simulink model "LOC_SYSTEM_20112024_2_Model"  (R2024a)
settings: Solver=VariableStepAuto  StartTime=0.0  StopTime=10.0  FixedStep=0.001  RelTol=1e-3
undefined symbols (not defined in the file): cp_oil, cp_water, engine_max_load, HE_heat_transfer_coefficient, HE_m1, HE_m2, HE_surface_area, HE_T1_ini, HE_T2_ini, LO_cooling_mass_oil_side, LO_cooling_mass_water_side, LO_heat_transfer_coefficient, LO_initial_temperatures
settings Model: ExtModeTrigDuration=100  Creator=ojklem  LastModifiedBy=ojklem
settings DataIOCC: StateSaveName=tmp_raccel_xout
settings OptimizationCC: EfficientMapNaN2IntZero=off
settings RTWCC: CustomBLASCallback=coder.internal.blas.MATLABBLASCallback
settings CodeAppCC: GenerateComments=off  MangleLength=10  SimulinkBlockComments=off

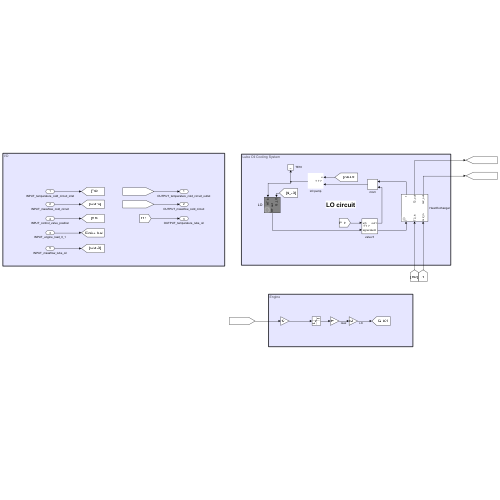
[thumbnail: Simulink's stored preview of the top-level diagram]
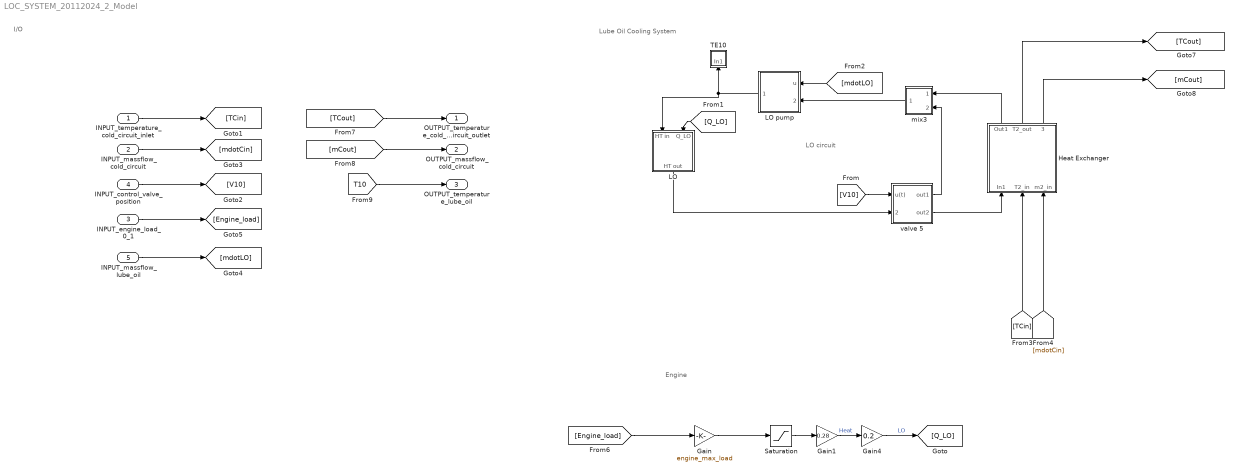
== system LOC_SYSTEM_20112024_2_Model ==
  note: LO circuit
  note: Lube Oil Cooling System
  note: Engine
  note: I/O
  INPUT_temperature_cold_circuit_inlet : Inport
  INPUT_massflow_cold_circuit : Inport  Port=2
  INPUT_engine_load_0_1 : Inport  Port=3
  INPUT_control_valve_position : Inport  Port=4
  INPUT_massflow_lube_oil : Inport  Port=5
  Gain : Gain  Gain=engine_max_load
  Gain1 : Gain  Gain=0.28
  Gain4 : Gain  Gain=0.2
  Heat Exchanger : Subsystem  mask{m1=HE_m1, m2=HE_m2, cp1=cp_water, cp2=cp_water, Tini=[HE_T1_ini, HE_T2_ini], A=HE_surface_area, h=HE_heat_transfer_coefficient}
      mask prompts: m1 "Mass side 1"; m2 "Mass side 2"; cp1 "Heat capacity side 1"; cp2 "Heat capacity side 2"; Tini "Initial value"; A "Area"; h "Heat transfer coefficient"
  LO : Subsystem  mask{K=LO_heat_transfer_coefficient, cpC=cp_water, cpSteel=cp_oil, MC=LO_cooling_mass_water_side, MSteel=LO_cooling_mass_oil_side, InitT=[LO_initial_temperatures, LO_initial_temperatures]}
      mask prompts: K "Heat transfer coefficient:"; cpC "Specific heat capacity water [J/kgK]:"; cpSteel "Specific heat capacity LO: [J/kgK]"; MC "Mass water [kg]:"; MSteel "Mass LO [kg]:"; InitT "Initial temperatures:"
  LO pump : Subsystem
      mask Display: image('pump.jpg');
  Saturation : Saturate  UpperLimit=engine_max_load  LowerLimit=0
  TE10 : Subsystem
  mix3 : Subsystem
      mask Display: % image('mix.png')
  valve 5 : Subsystem
      mask Display: image('valve3.png')
  OUTPUT_temperature_cold_circuit_outlet : Outport
  OUTPUT_massflow_cold_circuit : Outport  Port=2
  OUTPUT_temperature_lube_oil : Outport  Port=3
  wires:
  LO pump/1("  ") -> LO/1(HT in), TE10/1(In1)
  mix3/1(Out1) -> LO pump/2(" ")
  [mdotLO] -> LO pump/1(u)
  [mdotCin] -> Heat Exchanger/3(m2_in)
  [V10] -> valve 5/1(u(t))
  [TCin] -> Heat Exchanger/2(T2_in)
  Heat Exchanger/2(T2_out) -> [TCout]
  Heat Exchanger/1(Out1) -> mix3/1(In1)
  LO/1(HT out) -> valve 5/2(signal in)
  [Q_LO] -> LO/2(Q_LO)
  valve 5/2("out2 ") -> Heat Exchanger/1(In1)
  Heat Exchanger/3(m2_out) -> [mCout]
  valve 5/1(out1) -> mix3/2(In2)
  Gain1/1 -> Gain4/1  "Heat"
  Gain/1 -> Saturation/1
  [Engine_load] -> Gain/1
  Gain4/1 -> [Q_LO]  "LO"
  Saturation/1 -> Gain1/1
  [TCout] -> OUTPUT_temperature_cold_circuit_outlet/1
  INPUT_engine_load_0_1/1 -> [Engine_load]
  INPUT_massflow_cold_circuit/1 -> [mdotCin]
  INPUT_temperature_cold_circuit_inlet/1 -> [TCin]
  [mCout] -> OUTPUT_massflow_cold_circuit/1
  [T10] -> OUTPUT_temperature_lube_oil/1
  INPUT_control_valve_position/1 -> [V10]
  INPUT_massflow_lube_oil/1 -> [mdotLO]

== system LOC_SYSTEM_20112024_2_Model/Heat Exchanger ==
  In1 : Inport
  T2_in : Inport  Port=2
  m2_in : Inport  Port=3
  Demux : Demux  Outputs=2
  HX : Subsystem
      settings: PortSchema="{\"entries\":[{\"content\":{\"sides\":[{\"content\":{\"connectorIds\":[\"Out1\",\"Out2\",\"Out3\",\"Out4\"]},\"type\":\"ConnectorPlacement.EquallySpacedRectSide\",\"uuid\":\"b608803e-13f5-49cd-ab3a-92503d47ac52\"},{\"content\":{\"connectorIds\":[\"In1\",\"In2\",\"In3\",\"In4\"],\"side\":\"RIGHT\"},\"type\":\"ConnectorPlacement.EquallySpacedRectSide\",\"uuid\":\"cb859c45-d915-447d-9a89-62abad3e0c6f\"},{\"content\":{\"side\":\"TOP\"},\"type\":\"ConnectorPlacement.EquallySpacedRectSide\",\"uuid\":\"d365d95d-a075-458d-ace5-a17a7cf71809\"}]},\"type\":\"ConnectorPlacement.EquallySpacedConnector\",\"uuid\":\"ca673d01-47a6-46be-9ba4-be473b696b68\"}],\"packageUris\":[\"http://schema.mathworks.com/mf0/Connector/R2020b\"],\"version\":\"1.0\"}"
  Mux : Mux  Inputs=2
  Out1 : Outport
  T2_out : Outport  Port=2
  m2_out : Outport  Port=3
  wires:
  Demux/1 -> HX/4(T1_in)
  HX/4(T1_out) -> Mux/1
  Demux/2 -> HX/3(m1_in)
  HX/3(m1_out) -> Mux/2
  HX/1(m2_out) -> m2_out/1
  In1/1 -> Demux/1
  Mux/1 -> Out1/1
  T2_in/1 -> HX/2(T2_in)
  m2_in/1 -> HX/1(m2_in)
  HX/2(T2_out) -> T2_out/1

== system LOC_SYSTEM_20112024_2_Model/LO ==
  HT in : Inport
  Q_LO : Inport  Port=2
  Demux : Demux  Outputs=2
  Mux1 : Mux  Inputs=2
  Scope : Scope
  Subsystem : Subsystem
  Transport Delay : TransportDelay  Commented=on  DelayTime=0.2*60  InitialOutput=40
  Variable time-delay10 : Subsystem  Commented=on  mask{PipeVolume=MC/1000, InitOut=InitT(2)}
      mask prompts: PipeVolume "Pipe Volume [m^3]:"; InitOut "Initial Output:"
  HT out : Outport  VectorParamsAs1DForOutWhenUnconnected=off
  wires:
  Q_LO/1 -> Subsystem/3(Q)
  HT in/1 -> Demux/1
  Demux/2 -> Subsystem/2(m)
  Demux/1 -> Subsystem/1(Tin)
  Subsystem/3(m2) -> Mux1/2
  Subsystem/2(T) -> Scope/1
  Subsystem/1(Tout) -> Mux1/1
  Mux1/1 -> HT out/1

== system LOC_SYSTEM_20112024_2_Model/LO pump ==
  u : Inport
  " " : Inport  Port=2
  Demux : Demux  Outputs=2
  Mux8 : Mux  Inputs=2
  Scope : Scope
  "  " : Outport  VectorParamsAs1DForOutWhenUnconnected=off
  wires:
  " "/1 -> Demux/1
  Mux8/1 -> "  "/1
  u/1 -> Mux8/2
  Demux/2 -> Scope/1
  Demux/1 -> Mux8/1

== system LOC_SYSTEM_20112024_2_Model/TE10 ==
  In1 : Inport
  Gain : Gain  Gain=[1 0]  Multiplication=Matrix(K*u)
  tag scope: T10=global
  wires:
  Gain/1 -> [T10]
  In1/1 -> Gain/1

== system LOC_SYSTEM_20112024_2_Model/mix3 ==
  In1 : Inport
  In2 : Inport  Port=2
  Fcn : Fcn  Expr=(u(1)*u(2) + u(3)*u(4))/( u(2)+u(4) )
  Fcn1 : Fcn  Expr=u(2)+u(4)
  Mux1 : Mux  Inputs=2
  Mux2 : Mux  Inputs=2
  Scope1 : Scope
  Scope2 : Scope
  Out1 : Outport  VectorParamsAs1DForOutWhenUnconnected=off
  wires:
  In1/1 -> Scope1/1, Mux1/1
  Mux2/1 -> Out1/1
  In2/1 -> Mux1/2
  Fcn/1 -> Mux2/1
  Mux1/1 -> Fcn1/1, Scope2/1, Fcn/1
  Fcn1/1 -> Mux2/2

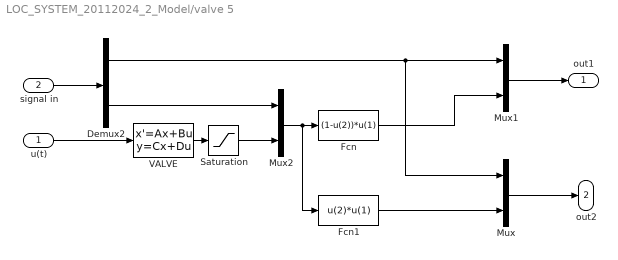
== system LOC_SYSTEM_20112024_2_Model/valve 5 ==
  u(t) : Inport
  signal in : Inport  Port=2
  Demux2 : Demux  Outputs=2
  Fcn : Fcn  Expr=(1-u(2))*u(1)
  Fcn1 : Fcn  Expr=u(2)*u(1)
  Mux : Mux  Inputs=2
  Mux1 : Mux  Inputs=2
  Mux2 : Mux  Inputs=2
  Saturation : Saturate  UpperLimit=0.99  LowerLimit=0.01
  VALVE : StateSpace  A=-1/1  B=1/1  D=0  InitialCondition=1
  out1 : Outport  VectorParamsAs1DForOutWhenUnconnected=off
  "out2 " : Outport  Port=2  VectorParamsAs1DForOutWhenUnconnected=off
  wires:
  Mux/1 -> "out2 "/1
  signal in/1 -> Demux2/1
  Mux1/1 -> out1/1
  Demux2/1 -> Mux/1, Mux1/1
  Mux2/1 -> Fcn1/1, Fcn/1
  Fcn/1 -> Mux1/2
  Fcn1/1 -> Mux/2
  VALVE/1 -> Saturation/1
  Demux2/2 -> Mux2/1
  u(t)/1 -> VALVE/1
  Saturation/1 -> Mux2/2

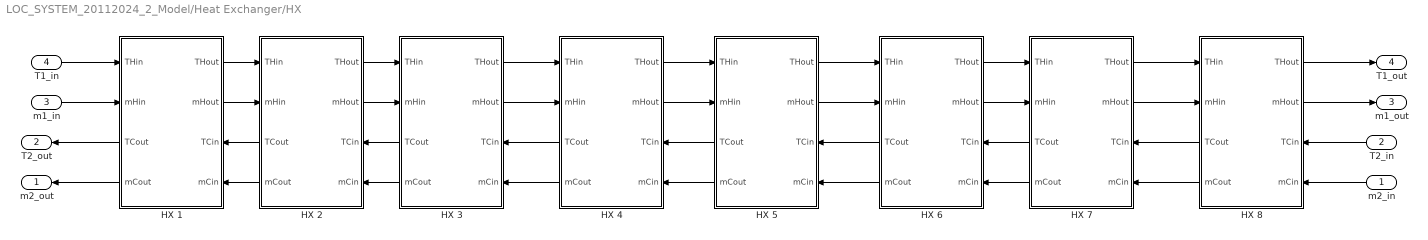
== system LOC_SYSTEM_20112024_2_Model/Heat Exchanger/HX ==
  m2_in : Inport
  T2_in : Inport  Port=2
  m1_in : Inport  Port=3
  T1_in : Inport  Port=4
  HX 1 : Subsystem
      settings: PortSchema="{\"entries\":[{\"content\":{\"sides\":[{\"content\":{\"connectorIds\":[\"In1\",\"In2\",\"Out3\",\"Out4\"]},\"type\":\"ConnectorPlacement.EquallySpacedRectSide\",\"uuid\":\"b608803e-13f5-49cd-ab3a-92503d47ac52\"},{\"content\":{\"connectorIds\":[\"Out1\",\"Out2\",\"In3\",\"In4\"],\"side\":\"RIGHT\"},\"type\":\"ConnectorPlacement.EquallySpacedRectSide\",\"uuid\":\"cb859c45-d915-447d-9a89-62abad3e0c6f\"},{\"content\":{\"connectorIds\":[],\"side\":\"TOP\"},\"type\":\"ConnectorPlacement.EquallySpacedRectSide\",\"uuid\":\"d365d95d-a075-458d-ace5-a17a7cf71809\"}]},\"type\":\"ConnectorPlacement.EquallySpacedConnector\",\"uuid\":\"ca673d01-47a6-46be-9ba4-be473b696b68\"}],\"packageUris\":[\"http://schema.mathworks.com/mf0/Connector/R2020b\"],\"version\":\"1.0\"}"
  HX 2 : Subsystem
      settings: PortSchema="{\"entries\":[{\"content\":{\"sides\":[{\"content\":{\"connectorIds\":[\"In1\",\"In2\",\"Out3\",\"Out4\"]},\"type\":\"ConnectorPlacement.EquallySpacedRectSide\",\"uuid\":\"b608803e-13f5-49cd-ab3a-92503d47ac52\"},{\"content\":{\"connectorIds\":[\"Out1\",\"Out2\",\"In3\",\"In4\"],\"side\":\"RIGHT\"},\"type\":\"ConnectorPlacement.EquallySpacedRectSide\",\"uuid\":\"cb859c45-d915-447d-9a89-62abad3e0c6f\"},{\"content\":{\"connectorIds\":[],\"side\":\"TOP\"},\"type\":\"ConnectorPlacement.EquallySpacedRectSide\",\"uuid\":\"d365d95d-a075-458d-ace5-a17a7cf71809\"}]},\"type\":\"ConnectorPlacement.EquallySpacedConnector\",\"uuid\":\"ca673d01-47a6-46be-9ba4-be473b696b68\"}],\"packageUris\":[\"http://schema.mathworks.com/mf0/Connector/R2020b\"],\"version\":\"1.0\"}"
  HX 3 : Subsystem
      settings: PortSchema="{\"entries\":[{\"content\":{\"sides\":[{\"content\":{\"connectorIds\":[\"In1\",\"In2\",\"Out3\",\"Out4\"]},\"type\":\"ConnectorPlacement.EquallySpacedRectSide\",\"uuid\":\"b608803e-13f5-49cd-ab3a-92503d47ac52\"},{\"content\":{\"connectorIds\":[\"Out1\",\"Out2\",\"In3\",\"In4\"],\"side\":\"RIGHT\"},\"type\":\"ConnectorPlacement.EquallySpacedRectSide\",\"uuid\":\"cb859c45-d915-447d-9a89-62abad3e0c6f\"},{\"content\":{\"connectorIds\":[],\"side\":\"TOP\"},\"type\":\"ConnectorPlacement.EquallySpacedRectSide\",\"uuid\":\"d365d95d-a075-458d-ace5-a17a7cf71809\"}]},\"type\":\"ConnectorPlacement.EquallySpacedConnector\",\"uuid\":\"ca673d01-47a6-46be-9ba4-be473b696b68\"}],\"packageUris\":[\"http://schema.mathworks.com/mf0/Connector/R2020b\"],\"version\":\"1.0\"}"
  HX 4 : Subsystem
      settings: PortSchema="{\"entries\":[{\"content\":{\"sides\":[{\"content\":{\"connectorIds\":[\"In1\",\"In2\",\"Out3\",\"Out4\"]},\"type\":\"ConnectorPlacement.EquallySpacedRectSide\",\"uuid\":\"b608803e-13f5-49cd-ab3a-92503d47ac52\"},{\"content\":{\"connectorIds\":[\"Out1\",\"Out2\",\"In3\",\"In4\"],\"side\":\"RIGHT\"},\"type\":\"ConnectorPlacement.EquallySpacedRectSide\",\"uuid\":\"cb859c45-d915-447d-9a89-62abad3e0c6f\"},{\"content\":{\"connectorIds\":[],\"side\":\"TOP\"},\"type\":\"ConnectorPlacement.EquallySpacedRectSide\",\"uuid\":\"d365d95d-a075-458d-ace5-a17a7cf71809\"}]},\"type\":\"ConnectorPlacement.EquallySpacedConnector\",\"uuid\":\"ca673d01-47a6-46be-9ba4-be473b696b68\"}],\"packageUris\":[\"http://schema.mathworks.com/mf0/Connector/R2020b\"],\"version\":\"1.0\"}"
  HX 5 : Subsystem
      settings: PortSchema="{\"entries\":[{\"content\":{\"sides\":[{\"content\":{\"connectorIds\":[\"In1\",\"In2\",\"Out3\",\"Out4\"]},\"type\":\"ConnectorPlacement.EquallySpacedRectSide\",\"uuid\":\"b608803e-13f5-49cd-ab3a-92503d47ac52\"},{\"content\":{\"connectorIds\":[\"Out1\",\"Out2\",\"In3\",\"In4\"],\"side\":\"RIGHT\"},\"type\":\"ConnectorPlacement.EquallySpacedRectSide\",\"uuid\":\"cb859c45-d915-447d-9a89-62abad3e0c6f\"},{\"content\":{\"connectorIds\":[],\"side\":\"TOP\"},\"type\":\"ConnectorPlacement.EquallySpacedRectSide\",\"uuid\":\"d365d95d-a075-458d-ace5-a17a7cf71809\"}]},\"type\":\"ConnectorPlacement.EquallySpacedConnector\",\"uuid\":\"ca673d01-47a6-46be-9ba4-be473b696b68\"}],\"packageUris\":[\"http://schema.mathworks.com/mf0/Connector/R2020b\"],\"version\":\"1.0\"}"
  HX 6 : Subsystem
      settings: PortSchema="{\"entries\":[{\"content\":{\"sides\":[{\"content\":{\"connectorIds\":[\"In1\",\"In2\",\"Out3\",\"Out4\"]},\"type\":\"ConnectorPlacement.EquallySpacedRectSide\",\"uuid\":\"b608803e-13f5-49cd-ab3a-92503d47ac52\"},{\"content\":{\"connectorIds\":[\"Out1\",\"Out2\",\"In3\",\"In4\"],\"side\":\"RIGHT\"},\"type\":\"ConnectorPlacement.EquallySpacedRectSide\",\"uuid\":\"cb859c45-d915-447d-9a89-62abad3e0c6f\"},{\"content\":{\"connectorIds\":[],\"side\":\"TOP\"},\"type\":\"ConnectorPlacement.EquallySpacedRectSide\",\"uuid\":\"d365d95d-a075-458d-ace5-a17a7cf71809\"}]},\"type\":\"ConnectorPlacement.EquallySpacedConnector\",\"uuid\":\"ca673d01-47a6-46be-9ba4-be473b696b68\"}],\"packageUris\":[\"http://schema.mathworks.com/mf0/Connector/R2020b\"],\"version\":\"1.0\"}"
  HX 7 : Subsystem
      settings: PortSchema="{\"entries\":[{\"content\":{\"sides\":[{\"content\":{\"connectorIds\":[\"In1\",\"In2\",\"Out3\",\"Out4\"]},\"type\":\"ConnectorPlacement.EquallySpacedRectSide\",\"uuid\":\"b608803e-13f5-49cd-ab3a-92503d47ac52\"},{\"content\":{\"connectorIds\":[\"Out1\",\"Out2\",\"In3\",\"In4\"],\"side\":\"RIGHT\"},\"type\":\"ConnectorPlacement.EquallySpacedRectSide\",\"uuid\":\"cb859c45-d915-447d-9a89-62abad3e0c6f\"},{\"content\":{\"connectorIds\":[],\"side\":\"TOP\"},\"type\":\"ConnectorPlacement.EquallySpacedRectSide\",\"uuid\":\"d365d95d-a075-458d-ace5-a17a7cf71809\"}]},\"type\":\"ConnectorPlacement.EquallySpacedConnector\",\"uuid\":\"ca673d01-47a6-46be-9ba4-be473b696b68\"}],\"packageUris\":[\"http://schema.mathworks.com/mf0/Connector/R2020b\"],\"version\":\"1.0\"}"
  HX 8 : Subsystem
      settings: PortSchema="{\"entries\":[{\"content\":{\"sides\":[{\"content\":{\"connectorIds\":[\"In1\",\"In2\",\"Out3\",\"Out4\"]},\"type\":\"ConnectorPlacement.EquallySpacedRectSide\",\"uuid\":\"b608803e-13f5-49cd-ab3a-92503d47ac52\"},{\"content\":{\"connectorIds\":[\"Out1\",\"Out2\",\"In3\",\"In4\"],\"side\":\"RIGHT\"},\"type\":\"ConnectorPlacement.EquallySpacedRectSide\",\"uuid\":\"cb859c45-d915-447d-9a89-62abad3e0c6f\"},{\"content\":{\"connectorIds\":[],\"side\":\"TOP\"},\"type\":\"ConnectorPlacement.EquallySpacedRectSide\",\"uuid\":\"d365d95d-a075-458d-ace5-a17a7cf71809\"}]},\"type\":\"ConnectorPlacement.EquallySpacedConnector\",\"uuid\":\"ca673d01-47a6-46be-9ba4-be473b696b68\"}],\"packageUris\":[\"http://schema.mathworks.com/mf0/Connector/R2020b\"],\"version\":\"1.0\"}"
  m2_out : Outport
  T2_out : Outport  Port=2
  m1_out : Outport  Port=3
  T1_out : Outport  Port=4
  wires:
  HX 1/4(mCout) -> m2_out/1
  m2_in/1 -> HX 8/4(mCin)
  HX 8/1(THout) -> T1_out/1
  HX 6/4(mCout) -> HX 5/4(mCin)
  HX 1/3(TCout) -> T2_out/1
  HX 8/4(mCout) -> HX 7/4(mCin)
  HX 7/2(mHout) -> HX 8/2(mHin)
  HX 8/3(TCout) -> HX 7/3(TCin)
  HX 7/1(THout) -> HX 8/1(THin)
  HX 4/4(mCout) -> HX 3/4(mCin)
  HX 6/3(TCout) -> HX 5/3(TCin)
  HX 4/3(TCout) -> HX 3/3(TCin)
  HX 3/1(THout) -> HX 4/1(THin)
  HX 5/1(THout) -> HX 6/1(THin)
  T1_in/1 -> HX 1/1(THin)
  HX 3/3(TCout) -> HX 2/3(TCin)
  T2_in/1 -> HX 8/3(TCin)
  HX 3/4(mCout) -> HX 2/4(mCin)
  HX 2/2(mHout) -> HX 3/2(mHin)
  HX 6/1(THout) -> HX 7/1(THin)
  HX 8/2(mHout) -> m1_out/1
  HX 6/2(mHout) -> HX 7/2(mHin)
  HX 3/2(mHout) -> HX 4/2(mHin)
  HX 7/3(TCout) -> HX 6/3(TCin)
  HX 7/4(mCout) -> HX 6/4(mCin)
  HX 5/2(mHout) -> HX 6/2(mHin)
  HX 2/4(mCout) -> HX 1/4(mCin)
  HX 5/4(mCout) -> HX 4/4(mCin)
  HX 1/2(mHout) -> HX 2/2(mHin)
  HX 2/1(THout) -> HX 3/1(THin)
  m1_in/1 -> HX 1/2(mHin)
  HX 5/3(TCout) -> HX 4/3(TCin)
  HX 1/1(THout) -> HX 2/1(THin)
  HX 4/2(mHout) -> HX 5/2(mHin)
  HX 4/1(THout) -> HX 5/1(THin)
  HX 2/3(TCout) -> HX 1/3(TCin)

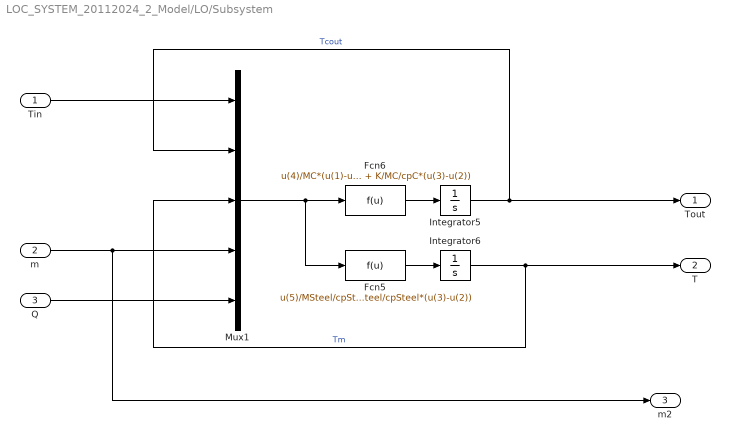
== system LOC_SYSTEM_20112024_2_Model/LO/Subsystem ==
  Tin : Inport
  m : Inport  Port=2
  Q : Inport  Port=3
  Fcn5 : Fcn  Expr=u(5)/MSteel/cpSteel - K/MSteel/cpSteel*(u(3)-u(2))
  Fcn6 : Fcn  Expr=u(4)/MC*(u(1)-u(2)) + K/MC/cpC*(u(3)-u(2))
  Integrator5 : Integrator  InitialCondition=InitT(1)
  Integrator6 : Integrator  InitialCondition=InitT(2)
  Mux1 : Mux  Inputs=5
  Tout : Outport  VectorParamsAs1DForOutWhenUnconnected=off
  T : Outport  Port=2  VectorParamsAs1DForOutWhenUnconnected=off
  m2 : Outport  Port=3  VectorParamsAs1DForOutWhenUnconnected=off
  wires:
  Q/1 -> Mux1/5
  Fcn6/1 -> Integrator5/1
  Integrator5/1 -> Tout/1, Mux1/2  "Tcout"
  m/1 -> m2/1, Mux1/4
  Mux1/1 -> Fcn5/1, Fcn6/1
  Fcn5/1 -> Integrator6/1
  Integrator6/1 -> T/1, Mux1/3  "Tm"
  Tin/1 -> Mux1/1

== system LOC_SYSTEM_20112024_2_Model/LO/Variable time-delay10 ==
  In1 : Inport
  Fcn : Fcn  Expr=1000*PipeVolume/u(1)
  Gain1 : Gain  Gain=[1 0]  Multiplication=Matrix(K*u) (u vector)
  Gain13 : Gain  Gain=[0 1]  Multiplication=Matrix(K*u) (u vector)
  Mux : Mux  Inputs=2
  Saturation : Saturate  UpperLimit=1000  LowerLimit=1
  Scope : Scope
  Variable Transport Delay : VariableTransportDelay  MaximumDelay=1000  InitialOutput=InitOut
  Out1 : Outport  VectorParamsAs1DForOutWhenUnconnected=off
  wires:
  Gain13/1 -> Fcn/1, Mux/2
  Mux/1 -> Out1/1
  Gain1/1 -> Variable Transport Delay/1
  Saturation/1 -> Variable Transport Delay/2, Scope/1
  Fcn/1 -> Saturation/1
  In1/1 -> Gain1/1, Gain13/1
  Variable Transport Delay/1 -> Mux/1

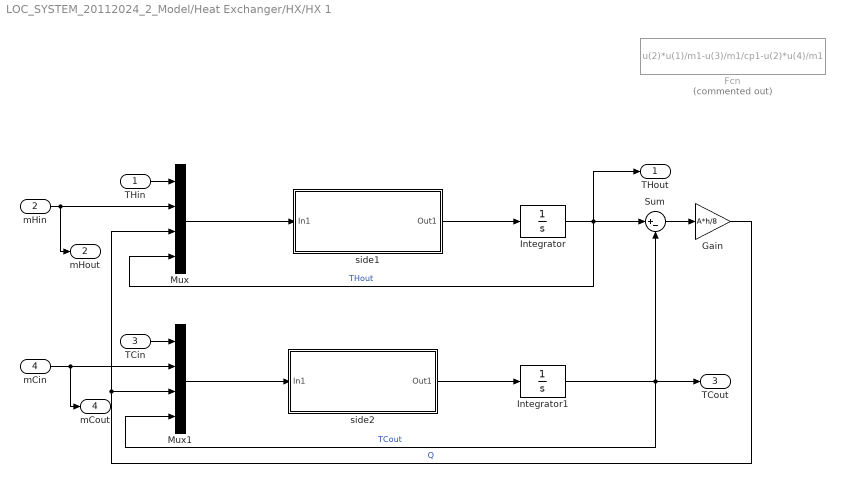
== system LOC_SYSTEM_20112024_2_Model/Heat Exchanger/HX/HX 1 ==
  THin : Inport
  mHin : Inport  Port=2
  TCin : Inport  Port=3
  mCin : Inport  Port=4
  Fcn : Fcn  Commented=on  Expr=u(2)*u(1)/m1-u(3)/m1/cp1-u(2)*u(4)/m1
  Gain : Gain  Gain=A*h/8
  Integrator : Integrator  InitialCondition=Tini(1)
  Integrator1 : Integrator  InitialCondition=Tini(2)
  Mux : Mux
  Mux1 : Mux
  Sum : Sum  Inputs=|+-
  side1 : Subsystem
  side2 : Subsystem
  THout : Outport  VectorParamsAs1DForOutWhenUnconnected=off
  mHout : Outport  Port=2  VectorParamsAs1DForOutWhenUnconnected=off
  TCout : Outport  Port=3  VectorParamsAs1DForOutWhenUnconnected=off
  mCout : Outport  Port=4  VectorParamsAs1DForOutWhenUnconnected=off
  wires:
  side1/1(Out1) -> Integrator/1
  Mux/1 -> side1/1(In1)
  mHin/1 -> mHout/1, Mux/2
  Gain/1 -> Mux/3, Mux1/3  "Q"
  THin/1 -> Mux/1
  TCin/1 -> Mux1/1
  mCin/1 -> mCout/1, Mux1/2
  Integrator1/1 -> Mux1/4, TCout/1, Sum/2  "TCout"
  side2/1(Out1) -> Integrator1/1
  Mux1/1 -> side2/1(In1)
  Sum/1 -> Gain/1
  Integrator/1 -> Mux/4, Sum/1, THout/1  "THout"

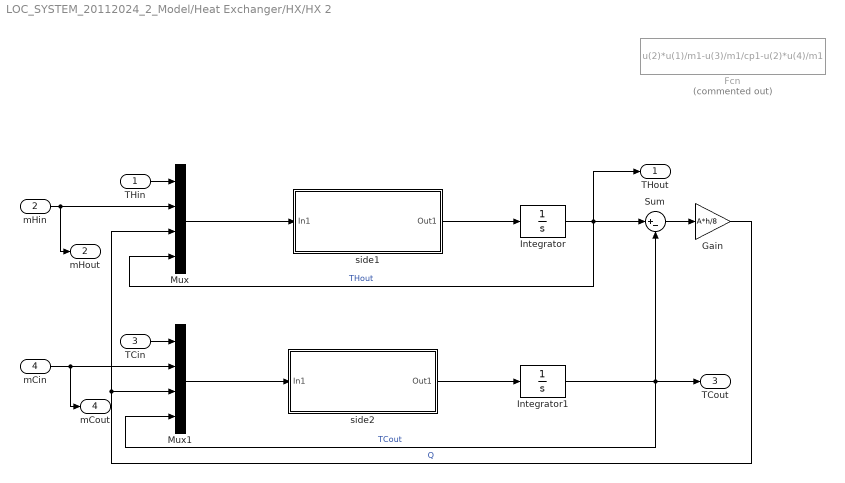
== system LOC_SYSTEM_20112024_2_Model/Heat Exchanger/HX/HX 2 ==
  THin : Inport
  mHin : Inport  Port=2
  TCin : Inport  Port=3
  mCin : Inport  Port=4
  Fcn : Fcn  Commented=on  Expr=u(2)*u(1)/m1-u(3)/m1/cp1-u(2)*u(4)/m1
  Gain : Gain  Gain=A*h/8
  Integrator : Integrator  InitialCondition=Tini(1)
  Integrator1 : Integrator  InitialCondition=Tini(2)
  Mux : Mux
  Mux1 : Mux
  Sum : Sum  Inputs=|+-
  side1 : Subsystem
  side2 : Subsystem
  THout : Outport  VectorParamsAs1DForOutWhenUnconnected=off
  mHout : Outport  Port=2  VectorParamsAs1DForOutWhenUnconnected=off
  TCout : Outport  Port=3  VectorParamsAs1DForOutWhenUnconnected=off
  mCout : Outport  Port=4  VectorParamsAs1DForOutWhenUnconnected=off
  wires:
  Integrator/1 -> THout/1, Sum/1, Mux/4  "THout"
  Sum/1 -> Gain/1
  Mux1/1 -> side2/1(In1)
  side2/1(Out1) -> Integrator1/1
  Integrator1/1 -> Sum/2, TCout/1, Mux1/4  "TCout"
  mCin/1 -> Mux1/2, mCout/1
  TCin/1 -> Mux1/1
  THin/1 -> Mux/1
  Gain/1 -> Mux1/3, Mux/3  "Q"
  mHin/1 -> Mux/2, mHout/1
  Mux/1 -> side1/1(In1)
  side1/1(Out1) -> Integrator/1

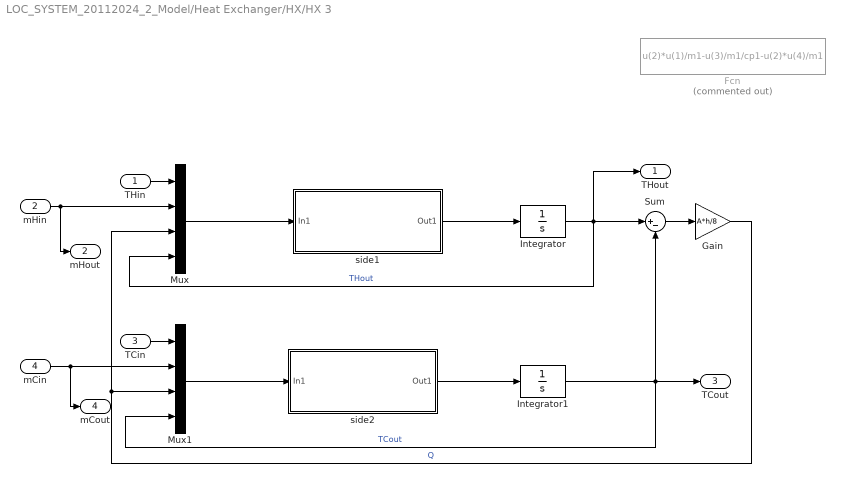
== system LOC_SYSTEM_20112024_2_Model/Heat Exchanger/HX/HX 3 ==
  THin : Inport
  mHin : Inport  Port=2
  TCin : Inport  Port=3
  mCin : Inport  Port=4
  Fcn : Fcn  Commented=on  Expr=u(2)*u(1)/m1-u(3)/m1/cp1-u(2)*u(4)/m1
  Gain : Gain  Gain=A*h/8
  Integrator : Integrator  InitialCondition=Tini(1)
  Integrator1 : Integrator  InitialCondition=Tini(2)
  Mux : Mux
  Mux1 : Mux
  Sum : Sum  Inputs=|+-
  side1 : Subsystem
  side2 : Subsystem
  THout : Outport  VectorParamsAs1DForOutWhenUnconnected=off
  mHout : Outport  Port=2  VectorParamsAs1DForOutWhenUnconnected=off
  TCout : Outport  Port=3  VectorParamsAs1DForOutWhenUnconnected=off
  mCout : Outport  Port=4  VectorParamsAs1DForOutWhenUnconnected=off
  wires:
  side1/1(Out1) -> Integrator/1
  Mux/1 -> side1/1(In1)
  mHin/1 -> mHout/1, Mux/2
  Gain/1 -> Mux/3, Mux1/3  "Q"
  THin/1 -> Mux/1
  TCin/1 -> Mux1/1
  mCin/1 -> mCout/1, Mux1/2
  Integrator1/1 -> Mux1/4, TCout/1, Sum/2  "TCout"
  side2/1(Out1) -> Integrator1/1
  Mux1/1 -> side2/1(In1)
  Sum/1 -> Gain/1
  Integrator/1 -> Mux/4, Sum/1, THout/1  "THout"

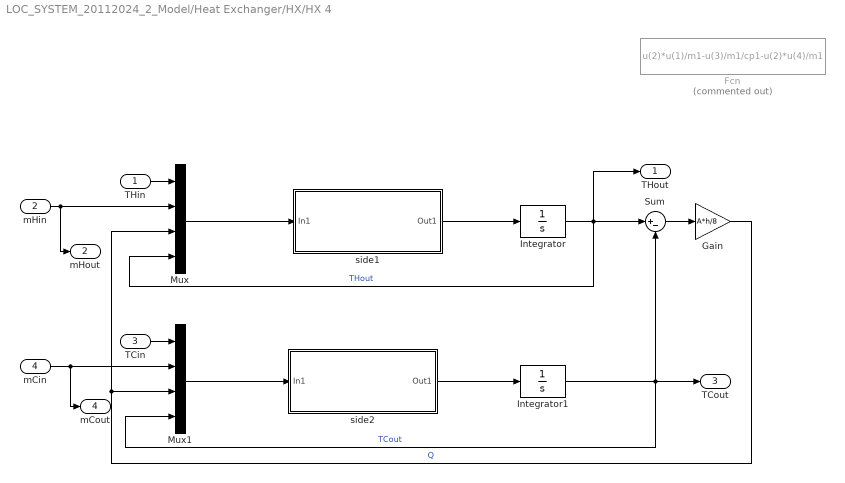
== system LOC_SYSTEM_20112024_2_Model/Heat Exchanger/HX/HX 4 ==
  THin : Inport
  mHin : Inport  Port=2
  TCin : Inport  Port=3
  mCin : Inport  Port=4
  Fcn : Fcn  Commented=on  Expr=u(2)*u(1)/m1-u(3)/m1/cp1-u(2)*u(4)/m1
  Gain : Gain  Gain=A*h/8
  Integrator : Integrator  InitialCondition=Tini(1)
  Integrator1 : Integrator  InitialCondition=Tini(2)
  Mux : Mux
  Mux1 : Mux
  Sum : Sum  Inputs=|+-
  side1 : Subsystem
  side2 : Subsystem
  THout : Outport  VectorParamsAs1DForOutWhenUnconnected=off
  mHout : Outport  Port=2  VectorParamsAs1DForOutWhenUnconnected=off
  TCout : Outport  Port=3  VectorParamsAs1DForOutWhenUnconnected=off
  mCout : Outport  Port=4  VectorParamsAs1DForOutWhenUnconnected=off
  wires:
  Integrator/1 -> THout/1, Sum/1, Mux/4  "THout"
  Sum/1 -> Gain/1
  Mux1/1 -> side2/1(In1)
  side2/1(Out1) -> Integrator1/1
  Integrator1/1 -> Sum/2, TCout/1, Mux1/4  "TCout"
  mCin/1 -> Mux1/2, mCout/1
  TCin/1 -> Mux1/1
  THin/1 -> Mux/1
  Gain/1 -> Mux1/3, Mux/3  "Q"
  mHin/1 -> Mux/2, mHout/1
  Mux/1 -> side1/1(In1)
  side1/1(Out1) -> Integrator/1

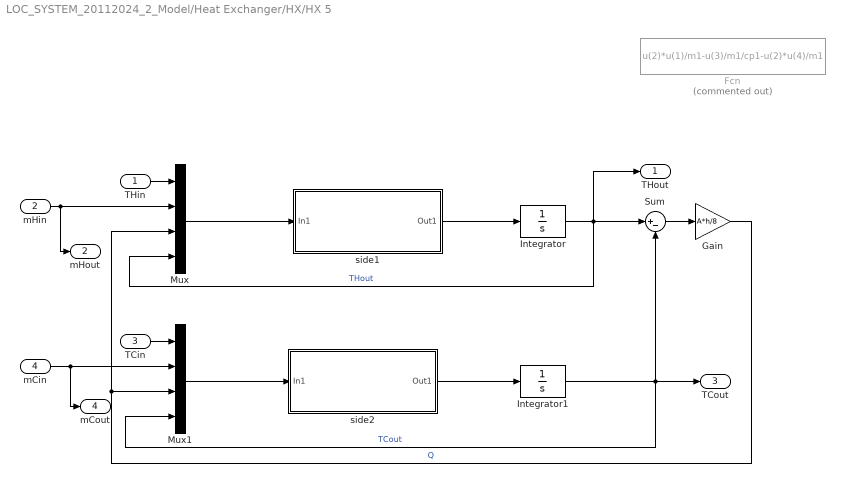
== system LOC_SYSTEM_20112024_2_Model/Heat Exchanger/HX/HX 5 ==
  THin : Inport
  mHin : Inport  Port=2
  TCin : Inport  Port=3
  mCin : Inport  Port=4
  Fcn : Fcn  Commented=on  Expr=u(2)*u(1)/m1-u(3)/m1/cp1-u(2)*u(4)/m1
  Gain : Gain  Gain=A*h/8
  Integrator : Integrator  InitialCondition=Tini(1)
  Integrator1 : Integrator  InitialCondition=Tini(2)
  Mux : Mux
  Mux1 : Mux
  Sum : Sum  Inputs=|+-
  side1 : Subsystem
  side2 : Subsystem
  THout : Outport  VectorParamsAs1DForOutWhenUnconnected=off
  mHout : Outport  Port=2  VectorParamsAs1DForOutWhenUnconnected=off
  TCout : Outport  Port=3  VectorParamsAs1DForOutWhenUnconnected=off
  mCout : Outport  Port=4  VectorParamsAs1DForOutWhenUnconnected=off
  wires:
  side1/1(Out1) -> Integrator/1
  Mux/1 -> side1/1(In1)
  mHin/1 -> mHout/1, Mux/2
  Gain/1 -> Mux/3, Mux1/3  "Q"
  THin/1 -> Mux/1
  TCin/1 -> Mux1/1
  mCin/1 -> mCout/1, Mux1/2
  Integrator1/1 -> Mux1/4, TCout/1, Sum/2  "TCout"
  side2/1(Out1) -> Integrator1/1
  Mux1/1 -> side2/1(In1)
  Sum/1 -> Gain/1
  Integrator/1 -> Mux/4, Sum/1, THout/1  "THout"

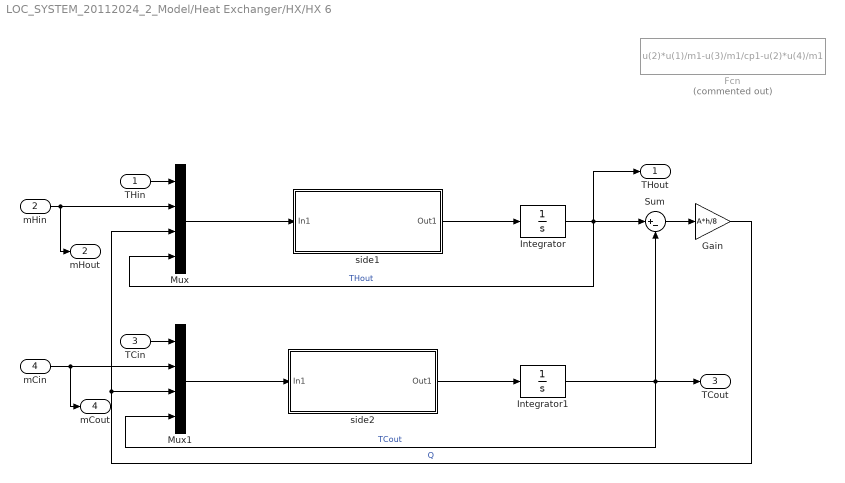
== system LOC_SYSTEM_20112024_2_Model/Heat Exchanger/HX/HX 6 ==
  THin : Inport
  mHin : Inport  Port=2
  TCin : Inport  Port=3
  mCin : Inport  Port=4
  Fcn : Fcn  Commented=on  Expr=u(2)*u(1)/m1-u(3)/m1/cp1-u(2)*u(4)/m1
  Gain : Gain  Gain=A*h/8
  Integrator : Integrator  InitialCondition=Tini(1)
  Integrator1 : Integrator  InitialCondition=Tini(2)
  Mux : Mux
  Mux1 : Mux
  Sum : Sum  Inputs=|+-
  side1 : Subsystem
  side2 : Subsystem
  THout : Outport  VectorParamsAs1DForOutWhenUnconnected=off
  mHout : Outport  Port=2  VectorParamsAs1DForOutWhenUnconnected=off
  TCout : Outport  Port=3  VectorParamsAs1DForOutWhenUnconnected=off
  mCout : Outport  Port=4  VectorParamsAs1DForOutWhenUnconnected=off
  wires:
  Integrator/1 -> THout/1, Sum/1, Mux/4  "THout"
  Sum/1 -> Gain/1
  Mux1/1 -> side2/1(In1)
  side2/1(Out1) -> Integrator1/1
  Integrator1/1 -> Sum/2, TCout/1, Mux1/4  "TCout"
  mCin/1 -> Mux1/2, mCout/1
  TCin/1 -> Mux1/1
  THin/1 -> Mux/1
  Gain/1 -> Mux1/3, Mux/3  "Q"
  mHin/1 -> Mux/2, mHout/1
  Mux/1 -> side1/1(In1)
  side1/1(Out1) -> Integrator/1

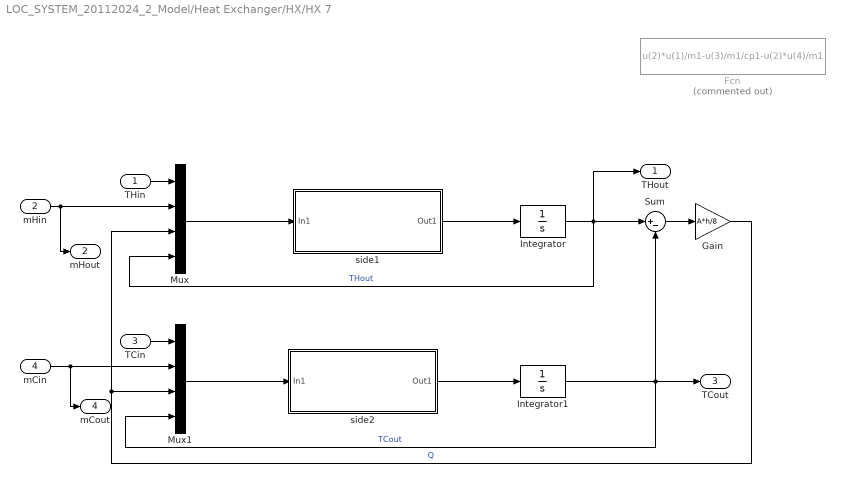
== system LOC_SYSTEM_20112024_2_Model/Heat Exchanger/HX/HX 7 ==
  THin : Inport
  mHin : Inport  Port=2
  TCin : Inport  Port=3
  mCin : Inport  Port=4
  Fcn : Fcn  Commented=on  Expr=u(2)*u(1)/m1-u(3)/m1/cp1-u(2)*u(4)/m1
  Gain : Gain  Gain=A*h/8
  Integrator : Integrator  InitialCondition=Tini(1)
  Integrator1 : Integrator  InitialCondition=Tini(2)
  Mux : Mux
  Mux1 : Mux
  Sum : Sum  Inputs=|+-
  side1 : Subsystem
  side2 : Subsystem
  THout : Outport  VectorParamsAs1DForOutWhenUnconnected=off
  mHout : Outport  Port=2  VectorParamsAs1DForOutWhenUnconnected=off
  TCout : Outport  Port=3  VectorParamsAs1DForOutWhenUnconnected=off
  mCout : Outport  Port=4  VectorParamsAs1DForOutWhenUnconnected=off
  wires:
  side1/1(Out1) -> Integrator/1
  Mux/1 -> side1/1(In1)
  mHin/1 -> mHout/1, Mux/2
  Gain/1 -> Mux/3, Mux1/3  "Q"
  THin/1 -> Mux/1
  TCin/1 -> Mux1/1
  mCin/1 -> mCout/1, Mux1/2
  Integrator1/1 -> Mux1/4, TCout/1, Sum/2  "TCout"
  side2/1(Out1) -> Integrator1/1
  Mux1/1 -> side2/1(In1)
  Sum/1 -> Gain/1
  Integrator/1 -> Mux/4, Sum/1, THout/1  "THout"

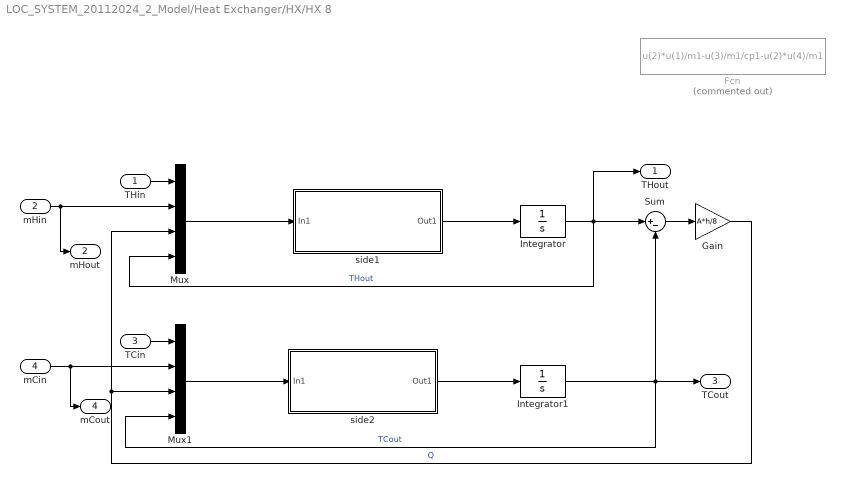
== system LOC_SYSTEM_20112024_2_Model/Heat Exchanger/HX/HX 8 ==
  THin : Inport
  mHin : Inport  Port=2
  TCin : Inport  Port=3
  mCin : Inport  Port=4
  Fcn : Fcn  Commented=on  Expr=u(2)*u(1)/m1-u(3)/m1/cp1-u(2)*u(4)/m1
  Gain : Gain  Gain=A*h/8
  Integrator : Integrator  InitialCondition=Tini(1)
  Integrator1 : Integrator  InitialCondition=Tini(2)
  Mux : Mux
  Mux1 : Mux
  Sum : Sum  Inputs=|+-
  side1 : Subsystem
  side2 : Subsystem
  THout : Outport  VectorParamsAs1DForOutWhenUnconnected=off
  mHout : Outport  Port=2  VectorParamsAs1DForOutWhenUnconnected=off
  TCout : Outport  Port=3  VectorParamsAs1DForOutWhenUnconnected=off
  mCout : Outport  Port=4  VectorParamsAs1DForOutWhenUnconnected=off
  wires:
  Integrator/1 -> THout/1, Sum/1, Mux/4  "THout"
  Sum/1 -> Gain/1
  Mux1/1 -> side2/1(In1)
  side2/1(Out1) -> Integrator1/1
  Integrator1/1 -> Sum/2, TCout/1, Mux1/4  "TCout"
  mCin/1 -> Mux1/2, mCout/1
  TCin/1 -> Mux1/1
  THin/1 -> Mux/1
  Gain/1 -> Mux1/3, Mux/3  "Q"
  mHin/1 -> Mux/2, mHout/1
  Mux/1 -> side1/1(In1)
  side1/1(Out1) -> Integrator/1

== system LOC_SYSTEM_20112024_2_Model/Heat Exchanger/HX/HX 1/side1 ==
  In1 : Inport
  Demux : Demux
  Gain1 : Gain  Gain=1/m1
  Gain2 : Gain  Gain=1/m1/cp1
  Gain3 : Gain  Gain=1/m1
  Product : Product
  Product1 : Product
  Sum1 : Sum  Inputs=+--
  Out1 : Outport
  wires:
  In1/1 -> Demux/1
  Sum1/1 -> Out1/1
  Gain1/1 -> Sum1/1
  Product/1 -> Gain1/1
  Gain3/1 -> Sum1/3  "Q"
  Demux/1 -> Product/1
  Demux/2 -> Product1/1, Product/2
  Gain2/1 -> Sum1/2  "Q"
  Product1/1 -> Gain3/1
  Demux/3 -> Gain2/1
  Demux/4 -> Product1/2

== system LOC_SYSTEM_20112024_2_Model/Heat Exchanger/HX/HX 1/side2 ==
  In1 : Inport
  Demux : Demux
  Gain1 : Gain  Gain=1/m2
  Gain2 : Gain  Gain=1/m2/cp2
  Gain3 : Gain  Gain=1/m2
  Product : Product
  Product1 : Product
  Sum1 : Sum  Inputs=++-
  Out1 : Outport
  wires:
  Demux/4 -> Product1/2
  Demux/3 -> Gain2/1
  Product1/1 -> Gain3/1
  Gain2/1 -> Sum1/2  "Q"
  Demux/2 -> Product/2, Product1/1
  Demux/1 -> Product/1
  Gain3/1 -> Sum1/3  "Q"
  Product/1 -> Gain1/1
  Gain1/1 -> Sum1/1
  Sum1/1 -> Out1/1
  In1/1 -> Demux/1

== system LOC_SYSTEM_20112024_2_Model/Heat Exchanger/HX/HX 2/side1 ==
  In1 : Inport
  Demux : Demux
  Gain1 : Gain  Gain=1/m1
  Gain2 : Gain  Gain=1/m1/cp1
  Gain3 : Gain  Gain=1/m1
  Product : Product
  Product1 : Product
  Sum1 : Sum  Inputs=+--
  Out1 : Outport
  wires:
  Demux/4 -> Product1/2
  Demux/3 -> Gain2/1
  Product1/1 -> Gain3/1
  Gain2/1 -> Sum1/2  "Q"
  Demux/2 -> Product/2, Product1/1
  Demux/1 -> Product/1
  Gain3/1 -> Sum1/3  "Q"
  Product/1 -> Gain1/1
  Gain1/1 -> Sum1/1
  Sum1/1 -> Out1/1
  In1/1 -> Demux/1

== system LOC_SYSTEM_20112024_2_Model/Heat Exchanger/HX/HX 2/side2 ==
  In1 : Inport
  Demux : Demux
  Gain1 : Gain  Gain=1/m2
  Gain2 : Gain  Gain=1/m2/cp2
  Gain3 : Gain  Gain=1/m2
  Product : Product
  Product1 : Product
  Sum1 : Sum  Inputs=++-
  Out1 : Outport
  wires:
  In1/1 -> Demux/1
  Sum1/1 -> Out1/1
  Gain1/1 -> Sum1/1
  Product/1 -> Gain1/1
  Gain3/1 -> Sum1/3  "Q"
  Demux/1 -> Product/1
  Demux/2 -> Product1/1, Product/2
  Gain2/1 -> Sum1/2  "Q"
  Product1/1 -> Gain3/1
  Demux/3 -> Gain2/1
  Demux/4 -> Product1/2

== system LOC_SYSTEM_20112024_2_Model/Heat Exchanger/HX/HX 3/side1 ==
  In1 : Inport
  Demux : Demux
  Gain1 : Gain  Gain=1/m1
  Gain2 : Gain  Gain=1/m1/cp1
  Gain3 : Gain  Gain=1/m1
  Product : Product
  Product1 : Product
  Sum1 : Sum  Inputs=+--
  Out1 : Outport
  wires:
  In1/1 -> Demux/1
  Sum1/1 -> Out1/1
  Gain1/1 -> Sum1/1
  Product/1 -> Gain1/1
  Gain3/1 -> Sum1/3  "Q"
  Demux/1 -> Product/1
  Demux/2 -> Product1/1, Product/2
  Gain2/1 -> Sum1/2  "Q"
  Product1/1 -> Gain3/1
  Demux/3 -> Gain2/1
  Demux/4 -> Product1/2

== system LOC_SYSTEM_20112024_2_Model/Heat Exchanger/HX/HX 3/side2 ==
  In1 : Inport
  Demux : Demux
  Gain1 : Gain  Gain=1/m2
  Gain2 : Gain  Gain=1/m2/cp2
  Gain3 : Gain  Gain=1/m2
  Product : Product
  Product1 : Product
  Sum1 : Sum  Inputs=++-
  Out1 : Outport
  wires:
  Demux/4 -> Product1/2
  Demux/3 -> Gain2/1
  Product1/1 -> Gain3/1
  Gain2/1 -> Sum1/2  "Q"
  Demux/2 -> Product/2, Product1/1
  Demux/1 -> Product/1
  Gain3/1 -> Sum1/3  "Q"
  Product/1 -> Gain1/1
  Gain1/1 -> Sum1/1
  Sum1/1 -> Out1/1
  In1/1 -> Demux/1

== system LOC_SYSTEM_20112024_2_Model/Heat Exchanger/HX/HX 4/side1 ==
  In1 : Inport
  Demux : Demux
  Gain1 : Gain  Gain=1/m1
  Gain2 : Gain  Gain=1/m1/cp1
  Gain3 : Gain  Gain=1/m1
  Product : Product
  Product1 : Product
  Sum1 : Sum  Inputs=+--
  Out1 : Outport
  wires:
  Demux/4 -> Product1/2
  Demux/3 -> Gain2/1
  Product1/1 -> Gain3/1
  Gain2/1 -> Sum1/2  "Q"
  Demux/2 -> Product/2, Product1/1
  Demux/1 -> Product/1
  Gain3/1 -> Sum1/3  "Q"
  Product/1 -> Gain1/1
  Gain1/1 -> Sum1/1
  Sum1/1 -> Out1/1
  In1/1 -> Demux/1

== system LOC_SYSTEM_20112024_2_Model/Heat Exchanger/HX/HX 4/side2 ==
  In1 : Inport
  Demux : Demux
  Gain1 : Gain  Gain=1/m2
  Gain2 : Gain  Gain=1/m2/cp2
  Gain3 : Gain  Gain=1/m2
  Product : Product
  Product1 : Product
  Sum1 : Sum  Inputs=++-
  Out1 : Outport
  wires:
  In1/1 -> Demux/1
  Sum1/1 -> Out1/1
  Gain1/1 -> Sum1/1
  Product/1 -> Gain1/1
  Gain3/1 -> Sum1/3  "Q"
  Demux/1 -> Product/1
  Demux/2 -> Product1/1, Product/2
  Gain2/1 -> Sum1/2  "Q"
  Product1/1 -> Gain3/1
  Demux/3 -> Gain2/1
  Demux/4 -> Product1/2

== system LOC_SYSTEM_20112024_2_Model/Heat Exchanger/HX/HX 5/side1 ==
  In1 : Inport
  Demux : Demux
  Gain1 : Gain  Gain=1/m1
  Gain2 : Gain  Gain=1/m1/cp1
  Gain3 : Gain  Gain=1/m1
  Product : Product
  Product1 : Product
  Sum1 : Sum  Inputs=+--
  Out1 : Outport
  wires:
  In1/1 -> Demux/1
  Sum1/1 -> Out1/1
  Gain1/1 -> Sum1/1
  Product/1 -> Gain1/1
  Gain3/1 -> Sum1/3  "Q"
  Demux/1 -> Product/1
  Demux/2 -> Product1/1, Product/2
  Gain2/1 -> Sum1/2  "Q"
  Product1/1 -> Gain3/1
  Demux/3 -> Gain2/1
  Demux/4 -> Product1/2

== system LOC_SYSTEM_20112024_2_Model/Heat Exchanger/HX/HX 5/side2 ==
  In1 : Inport
  Demux : Demux
  Gain1 : Gain  Gain=1/m2
  Gain2 : Gain  Gain=1/m2/cp2
  Gain3 : Gain  Gain=1/m2
  Product : Product
  Product1 : Product
  Sum1 : Sum  Inputs=++-
  Out1 : Outport
  wires:
  Demux/4 -> Product1/2
  Demux/3 -> Gain2/1
  Product1/1 -> Gain3/1
  Gain2/1 -> Sum1/2  "Q"
  Demux/2 -> Product/2, Product1/1
  Demux/1 -> Product/1
  Gain3/1 -> Sum1/3  "Q"
  Product/1 -> Gain1/1
  Gain1/1 -> Sum1/1
  Sum1/1 -> Out1/1
  In1/1 -> Demux/1

== system LOC_SYSTEM_20112024_2_Model/Heat Exchanger/HX/HX 6/side1 ==
  In1 : Inport
  Demux : Demux
  Gain1 : Gain  Gain=1/m1
  Gain2 : Gain  Gain=1/m1/cp1
  Gain3 : Gain  Gain=1/m1
  Product : Product
  Product1 : Product
  Sum1 : Sum  Inputs=+--
  Out1 : Outport
  wires:
  Demux/4 -> Product1/2
  Demux/3 -> Gain2/1
  Product1/1 -> Gain3/1
  Gain2/1 -> Sum1/2  "Q"
  Demux/2 -> Product/2, Product1/1
  Demux/1 -> Product/1
  Gain3/1 -> Sum1/3  "Q"
  Product/1 -> Gain1/1
  Gain1/1 -> Sum1/1
  Sum1/1 -> Out1/1
  In1/1 -> Demux/1

== system LOC_SYSTEM_20112024_2_Model/Heat Exchanger/HX/HX 6/side2 ==
  In1 : Inport
  Demux : Demux
  Gain1 : Gain  Gain=1/m2
  Gain2 : Gain  Gain=1/m2/cp2
  Gain3 : Gain  Gain=1/m2
  Product : Product
  Product1 : Product
  Sum1 : Sum  Inputs=++-
  Out1 : Outport
  wires:
  In1/1 -> Demux/1
  Sum1/1 -> Out1/1
  Gain1/1 -> Sum1/1
  Product/1 -> Gain1/1
  Gain3/1 -> Sum1/3  "Q"
  Demux/1 -> Product/1
  Demux/2 -> Product1/1, Product/2
  Gain2/1 -> Sum1/2  "Q"
  Product1/1 -> Gain3/1
  Demux/3 -> Gain2/1
  Demux/4 -> Product1/2

== system LOC_SYSTEM_20112024_2_Model/Heat Exchanger/HX/HX 7/side1 ==
  In1 : Inport
  Demux : Demux
  Gain1 : Gain  Gain=1/m1
  Gain2 : Gain  Gain=1/m1/cp1
  Gain3 : Gain  Gain=1/m1
  Product : Product
  Product1 : Product
  Sum1 : Sum  Inputs=+--
  Out1 : Outport
  wires:
  In1/1 -> Demux/1
  Sum1/1 -> Out1/1
  Gain1/1 -> Sum1/1
  Product/1 -> Gain1/1
  Gain3/1 -> Sum1/3  "Q"
  Demux/1 -> Product/1
  Demux/2 -> Product1/1, Product/2
  Gain2/1 -> Sum1/2  "Q"
  Product1/1 -> Gain3/1
  Demux/3 -> Gain2/1
  Demux/4 -> Product1/2

== system LOC_SYSTEM_20112024_2_Model/Heat Exchanger/HX/HX 7/side2 ==
  In1 : Inport
  Demux : Demux
  Gain1 : Gain  Gain=1/m2
  Gain2 : Gain  Gain=1/m2/cp2
  Gain3 : Gain  Gain=1/m2
  Product : Product
  Product1 : Product
  Sum1 : Sum  Inputs=++-
  Out1 : Outport
  wires:
  Demux/4 -> Product1/2
  Demux/3 -> Gain2/1
  Product1/1 -> Gain3/1
  Gain2/1 -> Sum1/2  "Q"
  Demux/2 -> Product/2, Product1/1
  Demux/1 -> Product/1
  Gain3/1 -> Sum1/3  "Q"
  Product/1 -> Gain1/1
  Gain1/1 -> Sum1/1
  Sum1/1 -> Out1/1
  In1/1 -> Demux/1

== system LOC_SYSTEM_20112024_2_Model/Heat Exchanger/HX/HX 8/side1 ==
  In1 : Inport
  Demux : Demux
  Gain1 : Gain  Gain=1/m1
  Gain2 : Gain  Gain=1/m1/cp1
  Gain3 : Gain  Gain=1/m1
  Product : Product
  Product1 : Product
  Sum1 : Sum  Inputs=+--
  Out1 : Outport
  wires:
  Demux/4 -> Product1/2
  Demux/3 -> Gain2/1
  Product1/1 -> Gain3/1
  Gain2/1 -> Sum1/2  "Q"
  Demux/2 -> Product/2, Product1/1
  Demux/1 -> Product/1
  Gain3/1 -> Sum1/3  "Q"
  Product/1 -> Gain1/1
  Gain1/1 -> Sum1/1
  Sum1/1 -> Out1/1
  In1/1 -> Demux/1

== system LOC_SYSTEM_20112024_2_Model/Heat Exchanger/HX/HX 8/side2 ==
  In1 : Inport
  Demux : Demux
  Gain1 : Gain  Gain=1/m2
  Gain2 : Gain  Gain=1/m2/cp2
  Gain3 : Gain  Gain=1/m2
  Product : Product
  Product1 : Product
  Sum1 : Sum  Inputs=++-
  Out1 : Outport
  wires:
  In1/1 -> Demux/1
  Sum1/1 -> Out1/1
  Gain1/1 -> Sum1/1
  Product/1 -> Gain1/1
  Gain3/1 -> Sum1/3  "Q"
  Demux/1 -> Product/1
  Demux/2 -> Product1/1, Product/2
  Gain2/1 -> Sum1/2  "Q"
  Product1/1 -> Gain3/1
  Demux/3 -> Gain2/1
  Demux/4 -> Product1/2
